simulink model "TestFuzzy"  (R2018a)
settings: Solver=VariableStepAuto  StartTime=0.0  StopTime=30  RelTol=1e-3
libraries: fuzblock x1
settings Model: Creator=egydi  LastModifiedBy=egydi

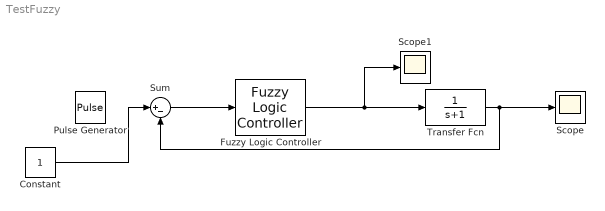
== system TestFuzzy ==
  Constant : Constant
  Fuzzy Logic Controller : fuzblock/Fuzzy Logic  Controller  FIS='HelloWorld.fis'  OutputSampleNumber=101  DataType=double  FuzzifiedInputs=off  RuleFiringStrengths=off  RuleOutputs=off  AggregatedOutputs=off  SimulateUsing=Interpreted execution  OutOfRangeInputValueMessage=warning  NoRuleFiredMessage=warning  EmptyOutputFuzzySetMessage=warning
  Pulse Generator : DiscretePulseGenerator  PulseType=Time based  Period=20  PulseWidth=50
  Scope : Scope
  Scope1 : Scope
  Sum : Sum  Inputs=|+-
  Transfer Fcn : TransferFcn  Denominator=[1 1]
  wires:
  Fuzzy Logic Controller/1 -> Scope1/1, Transfer Fcn/1
  Sum/1 -> Fuzzy Logic Controller/1
  Transfer Fcn/1 -> Scope/1, Sum/2
  Constant/1 -> Sum/1
